simulink model "Visualizer"  (R2015b)
settings: Solver=FixedStepDiscrete  StartTime=0.0  StopTime=Time  FixedStep=Ts  RelTol=1e-3
undefined symbols (not defined in the file or in its folder): quad
libraries: realtime_pacer_lib x2, simulink x1
settings Model: SimulationMode=accelerator  Creator=Carlos  LastModifiedBy=carlosluis
settings DataIOCC: SaveFormat=Array
settings DebuggingCC: UnderspecifiedInitializationDetection=Classic  MergeDetectMultiDrivingBlocksExec=none  SolverPrmCheckMsg=warning  MultiTaskRateTransMsg=warning  StateNameClashWarn=warning
settings HardwareCC: ProdBitPerPointer=32  ProdLargestAtomicFloat=None  ProdIntDivRoundTo=Undefined  ProdEndianess=Unspecified  ProdWordSize=32  ProdHWDeviceType=32-bit Generic
settings GRTTargetCC: GeneratePreprocessorConditionals=Disable all
settings ConfigComp: CovModelRefEnable=Off

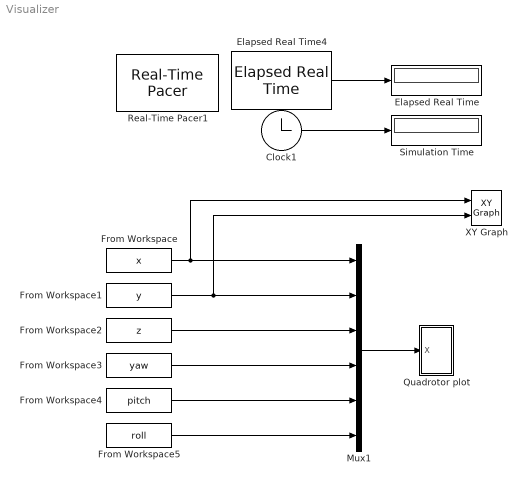
== system Visualizer ==
  Clock1 : Clock
  Elapsed Real Time : Display
      settings: Decimation=2
  Elapsed Real Time4 : realtime_pacer_lib/Elapsed Real Time
  From Workspace : FromWorkspace  VariableName=x
  From Workspace1 : FromWorkspace  VariableName=y
  From Workspace2 : FromWorkspace  VariableName=z
  From Workspace3 : FromWorkspace  VariableName=yaw
  From Workspace4 : FromWorkspace  VariableName=pitch
  From Workspace5 : FromWorkspace  VariableName=roll
  Mux1 : Mux  Inputs=6
  Quadrotor plot : Subsystem  AncestorBlock=roblocks/Robot Graphics/Quadrotor plot  mask{quad=quad, xydim=2, zdim=2.3}
      mask prompts: quad "Model"; xydim "xy-axes dimension"; zdim "z-axis dimension"
      mask help: Animate quadrotor.
      mask Help:
      | This block graphically displays a quadrotor (flying robot).
      | 
      | A new figure is created and A graphical model of a quadrotor is animated
      | to a pose specified by the state vector input to the block.
      | 
      | The state vector is [x y z roll pitch yaw] in world coordinates and the
      | angles are in radians.
      | 
      | Notes:
      | - The dimensions of the vehicle workspace are set by parameters
  Real-Time Pacer1 : realtime_pacer_lib/Real-Time Pacer  simTimePerRealTime=1
  Simulation Time : Display
      settings: Decimation=2
  XY Graph : simulink/Sinks/XY Graph  xmin=-2  xmax=2  ymin=-2  ymax=2  st=Ts
  wires:
  Mux1/1 -> Quadrotor plot/1(X)
  From Workspace/1 -> XY Graph/1, Mux1/1
  From Workspace1/1 -> XY Graph/2, Mux1/2
  From Workspace2/1 -> Mux1/3
  From Workspace3/1 -> Mux1/4
  From Workspace4/1 -> Mux1/5
  From Workspace5/1 -> Mux1/6
  Elapsed Real Time4/1 -> Elapsed Real Time/1
  Clock1/1 -> Simulation Time/1

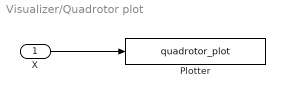
== system Visualizer/Quadrotor plot ==
  X : Inport
  Plotter : S-Function  FunctionName=quadrotor_plot  Parameters=[xydim, zdim], 1, 1,quad  SFunctionDeploymentMode=off  EnableBusSupport=off
  wires:
  X/1 -> Plotter/1
